simulink model "Simulink_bouncinng_ball"  (R2025b)
settings: Solver=VariableStepAuto  StartTime=0.0  StopTime=10.0  RelTol=1e-3
settings Model: Creator=leonard  LastModifiedBy=leonard

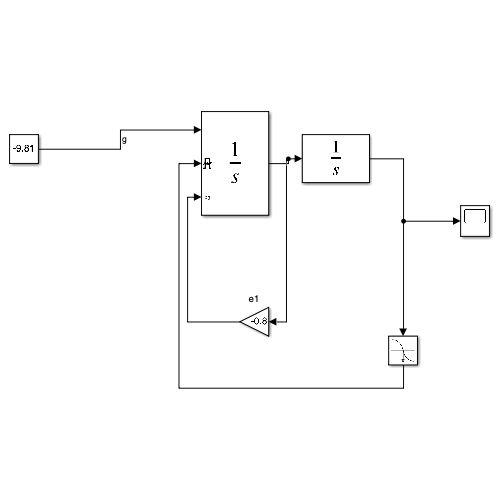
[thumbnail: Simulink's stored preview of the top-level diagram]
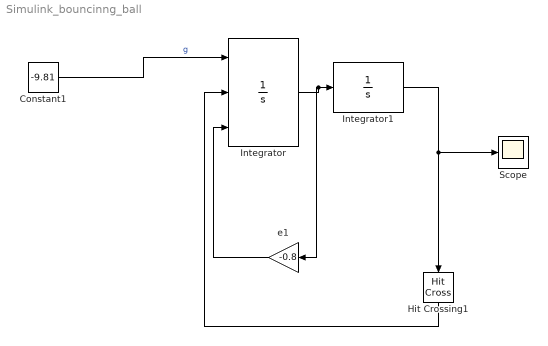
== system Simulink_bouncinng_ball ==
  Constant1 : Constant  Value=-9.81
  Hit Crossing1 : HitCross  HitCrossingDirection=falling
  Integrator : Integrator  ExternalReset=either  InitialConditionSource=external
  Integrator1 : Integrator  InitialCondition=2
  Scope : Scope
      settings: ActiveDisplayYMinimum=-2.8632868669174107  ActiveDisplayYMaximum=5.9404776892175386
  e1 : Gain  Gain=-0.8
  wires:
  Constant1/1 -> Integrator/1  "g"
  Integrator1/1 -> Scope/1, Hit Crossing1/1
  Integrator/1 -> e1/1, Integrator1/1
  Hit Crossing1/1 -> Integrator/2
  e1/1 -> Integrator/3
